simulink model "fir_filter"  (R2020a)
settings: Solver=VariableStepAuto  StartTime=0.0  StopTime=10.0  RelTol=1e-3
settings Model: Creator=Shubham  LastModifiedBy=Shubham

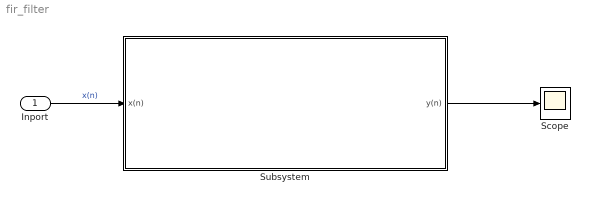
== system fir_filter ==
  Inport : Inport
  Scope : Scope
  Subsystem : Subsystem
  wires:
  Inport/1 -> Subsystem/1(x(n))  "x(n)"
  Subsystem/1(y(n)) -> Scope/1

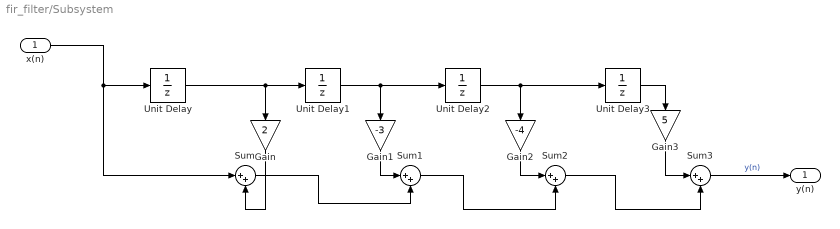
== system fir_filter/Subsystem ==
  x(n) : Inport
  Gain : Gain  Gain=2
  Gain1 : Gain  Gain=-3
  Gain2 : Gain  Gain=-4
  Gain3 : Gain  Gain=5
  Sum{,1..3} (4 alike) : Sum  Inputs=|++
  Unit Delay{,1..3} (4 alike) : UnitDelay  SampleTime=-1  HasFrameUpgradeWarning=on
  y(n) : Outport
  wires:
  Gain/1 -> Sum/2
  Sum2/1 -> Sum3/2
  Unit Delay1/1 -> Gain1/1, Unit Delay2/1
  Unit Delay2/1 -> Unit Delay3/1, Gain2/1
  x(n)/1 -> Sum/1, Unit Delay/1
  Sum1/1 -> Sum2/2
  Gain3/1 -> Sum3/1
  Unit Delay/1 -> Gain/1, Unit Delay1/1
  Unit Delay3/1 -> Gain3/1
  Gain1/1 -> Sum1/1
  Gain2/1 -> Sum2/1
  Sum/1 -> Sum1/2
  Sum3/1 -> y(n)/1  "y(n)"
